simulink model "mobileRobotSimulink"  (R2018b)
settings: Solver=VariableStepAuto  StartTime=0.0  StopTime=350  RelTol=1e-3
libraries: simulink x1
settings Model: PauseTimes=50  Creator=Mohsen  LastModifiedBy=Mohsen

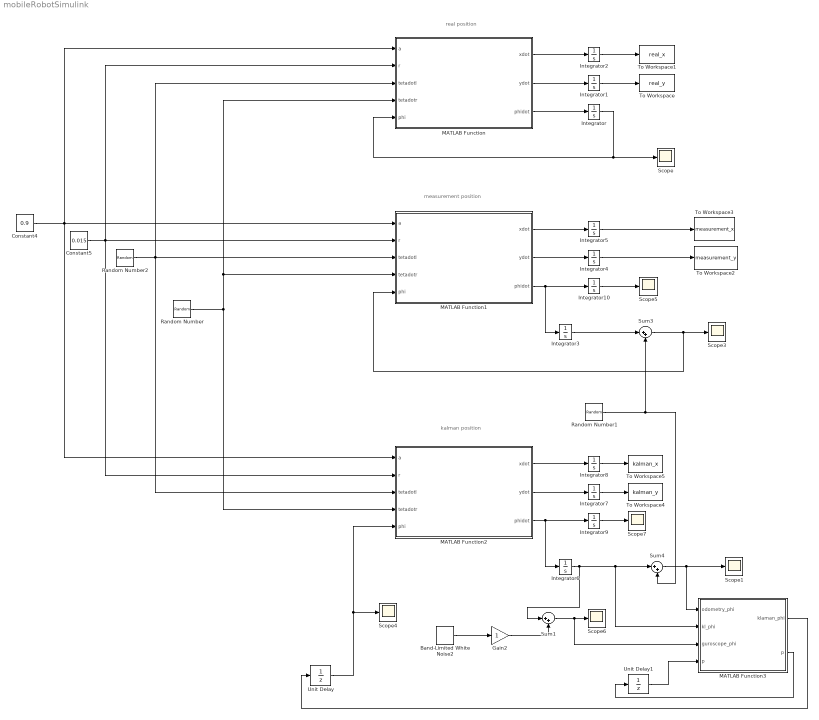
== system mobileRobotSimulink ==
  note: real position
  note: measurement position
  note: kalman position
  Band-Limited White Noise2 : simulink/Sources/Band-Limited White Noise  Cov=[0.00001]  Ts=0.01  seed=[23341]
  Constant4 : Constant  Value=0.9
  Constant5 : Constant  Value=0.015
  Gain2 : Gain
  Integrator{,1..10} (11 alike) : Integrator
  MATLAB Function : MATLAB Function  TreatAsAtomicUnit=on
  MATLAB Function1 : MATLAB Function  TreatAsAtomicUnit=on
  MATLAB Function2 : MATLAB Function  TreatAsAtomicUnit=on
  MATLAB Function3 : MATLAB Function  TreatAsAtomicUnit=on
  Random Number : RandomNumber  Mean=1  Variance=2  SampleTime=0.1
  Random Number1 : RandomNumber  Mean=0.05  Variance=0.1  SampleTime=0.1
  Random Number2 : RandomNumber  Mean=0.05  Variance=1.5  SampleTime=0.1
  Scope{,1,3..7} (7 alike) : Scope
  Sum1 : Sum  Inputs=|++
  Sum3 : Sum  Inputs=|++
  Sum4 : Sum  Inputs=|++
  To Workspace : ToWorkspace  VariableName=real_y  SaveFormat=Structure With Time  SampleTime=-1
      settings: StopFcn=rob_plot3(real_x.signals.values,real_y.signals.values,measurement_x.signals.values,measurement_y.signals.values,kalman_x.signals.values,kalman_y.signals.values)
  To Workspace1 : ToWorkspace  VariableName=real_x  SaveFormat=Structure With Time  SampleTime=-1
      settings: StopFcn=rob_plot3(real_x.signals.values,real_y.signals.values,measurement_x.signals.values,measurement_y.signals.values,kalman_x.signals.values,kalman_y.signals.values)
  To Workspace2 : ToWorkspace  VariableName=measurement_y  SaveFormat=Structure With Time  SampleTime=-1
      settings: StopFcn=rob_plot3(real_x.signals.values,real_y.signals.values,measurement_x.signals.values,measurement_y.signals.values,kalman_x.signals.values,kalman_y.signals.values)
  To Workspace3 : ToWorkspace  VariableName=measurement_x  SaveFormat=Structure With Time  SampleTime=-1
      settings: StopFcn=rob_plot3(real_x.signals.values,real_y.signals.values,measurement_x.signals.values,measurement_y.signals.values,kalman_x.signals.values,kalman_y.signals.values)
  To Workspace4 : ToWorkspace  VariableName=kalman_y  SaveFormat=Structure With Time  SampleTime=-1
      settings: StopFcn=rob_plot3(real_x.signals.values,real_y.signals.values,measurement_x.signals.values,measurement_y.signals.values,kalman_x.signals.values,kalman_y.signals.values)
  To Workspace5 : ToWorkspace  VariableName=kalman_x  SaveFormat=Structure With Time  SampleTime=-1
      settings: StopFcn=rob_plot3(real_x.signals.values,real_y.signals.values,measurement_x.signals.values,measurement_y.signals.values,kalman_x.signals.values,kalman_y.signals.values)
  Unit Delay : UnitDelay  SampleTime=-1
  Unit Delay1 : UnitDelay  SampleTime=-1
  wires:
  MATLAB Function/3(phidot) -> Integrator/1
  MATLAB Function/1(xdot) -> Integrator2/1
  MATLAB Function/2(ydot) -> Integrator1/1
  Integrator2/1 -> To Workspace1/1
  Integrator1/1 -> To Workspace/1
  Integrator/1 -> MATLAB Function/5(phi), Scope/1
  Sum3/1 -> Scope3/1, MATLAB Function1/5(phi)
  Random Number1/1 -> Sum4/2, Sum3/2
  MATLAB Function1/1(xdot) -> Integrator5/1
  MATLAB Function1/2(ydot) -> Integrator4/1
  Integrator4/1 -> To Workspace2/1
  Integrator5/1 -> To Workspace3/1
  MATLAB Function1/3(phidot) -> Integrator10/1, Integrator3/1
  Integrator3/1 -> Sum3/1
  Constant5/1 -> MATLAB Function/2(r), MATLAB Function1/2(r), MATLAB Function2/2(r)
  Integrator6/1 -> Sum1/1, MATLAB Function3/2(kl_phi), Sum4/1
  MATLAB Function2/3(phidot) -> Integrator9/1, Integrator6/1
  Constant4/1 -> MATLAB Function1/1(a), MATLAB Function2/1(a), MATLAB Function/1(a)
  Sum1/1 -> MATLAB Function3/3(guroscope_phi), Scope6/1
  MATLAB Function2/2(ydot) -> Integrator7/1
  Integrator7/1 -> To Workspace4/1
  Integrator8/1 -> To Workspace5/1
  Random Number2/1 -> MATLAB Function2/3(tetadotl), MATLAB Function/3(tetadotl), MATLAB Function1/3(tetadotl)
  Sum4/1 -> MATLAB Function3/1(odometry_phi), Scope1/1
  Gain2/1 -> Sum1/2
  MATLAB Function2/1(xdot) -> Integrator8/1
  Random Number/1 -> MATLAB Function/4(tetadotr), MATLAB Function1/4(tetadotr), MATLAB Function2/4(tetadotr)
  MATLAB Function3/1(klaman_phi) -> Unit Delay/1
  MATLAB Function3/2(p) -> Unit Delay1/1
  Unit Delay1/1 -> MATLAB Function3/4("p ")
  Band-Limited White Noise2/1 -> Gain2/1
  Unit Delay/1 -> Scope4/1, MATLAB Function2/5(phi)
  Integrator9/1 -> Scope7/1
  Integrator10/1 -> Scope5/1

== matlab function mobileRobotSimulink/MATLAB Function1 ==
  data: a input; r input; tetadotl input; xdot output; ydot output; phidot output; tetadotr input; phi input
function [xdot, ydot, phidot] = fcn(a, r, tetadotl, tetadotr, phi)

xdot = (r/2)*(tetadotr*cos(phi)+tetadotl*cos(phi));
ydot = (r/2)*(tetadotr*sin(phi)+tetadotl*sin(phi));
phidot = (r/(2*a))*(tetadotr-tetadotl);

== matlab function mobileRobotSimulink/MATLAB Function ==
  data: a input; r input; tetadotl input; xdot output; ydot output; phidot output; tetadotr input; phi input
function [xdot, ydot, phidot] = fcn(a, r, tetadotl, tetadotr, phi)

xdot = (r/2)*(tetadotr*cos(phi)+tetadotl*cos(phi));
ydot = (r/2)*(tetadotr*sin(phi)+tetadotl*sin(phi));
phidot = (r/(2*a))*(tetadotr-tetadotl);

== matlab function mobileRobotSimulink/MATLAB Function2 ==
  data: a input; r input; tetadotl input; xdot output; ydot output; phidot output; tetadotr input; phi input
function [xdot, ydot, phidot] = fcn(a, r, tetadotl, tetadotr, phi)

xdot = (r/2)*(tetadotr*cos(phi)+tetadotl*cos(phi));
ydot = (r/2)*(tetadotr*sin(phi)+tetadotl*sin(phi));
phidot = (r/(2*a))*(tetadotr-tetadotl);

== matlab function mobileRobotSimulink/MATLAB Function3 ==
  data: klaman_phi output; p output; odometry_phi input; kl_phi input; guroscope_phi input; p input
function [klaman_phi,p]= fcn(odometry_phi, kl_phi, guroscope_phi, p)

processNoise     = 0.5;
gyroscope_noise = 0.1;

%-------------------- "Prediction Step" --------------------
u = odometry_phi; 
kl_phi = kl_phi + u; 
p = p + processNoise;

%-------------------- "Update Step" --------------------
z = guroscope_phi;
y = z - kl_phi;                        

k = p / (p + gyroscope_noise);  
klaman_phi = kl_phi + (k * y);                   
p = (1 - k)*p;
